simulink model "practical_class_2_2b_simulink"  (R2023b)
settings: Solver=VariableStepAuto  StartTime=0.0  StopTime=30  RelTol=1e-3
values from neighbouring files (symbols this model uses):
  b1 = 8    [practical_class_2_2b.m]
  b2 = 7    [practical_class_2_2b.m]
  k1 = 2    [practical_class_2_2b.m]
  k2 = 4    [practical_class_2_2b.m]
  m1 = 4    [practical_class_2_2b.m]
  m2 = 2    [practical_class_2_2b.m]
settings Model: Creator=klysm  LastModifiedBy=klysm

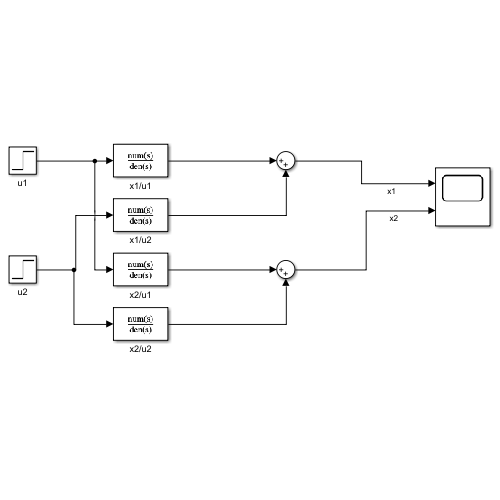
[thumbnail: Simulink's stored preview of the top-level diagram]
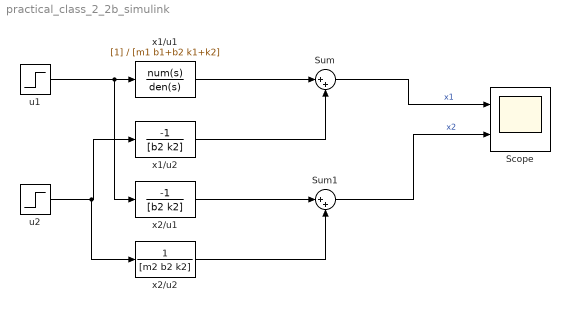
== system practical_class_2_2b_simulink ==
  Scope : Scope  NumInputPorts=2
  Sum : Sum  Inputs=|++
  Sum1 : Sum  Inputs=|++
  u1 : Step  Time=2  SampleTime=0
  u2 : Step  Time=10  After=0.7  SampleTime=0
  x1/u1 : TransferFcn  Denominator=[m1 b1+b2 k1+k2]
  x1/u2 : TransferFcn  Numerator=[-1]  Denominator=[b2 k2]
  x2/u1 : TransferFcn  Numerator=[-1]  Denominator=[b2 k2]
  x2/u2 : TransferFcn  Denominator=[m2 b2 k2]
  wires:
  Sum/1 -> Scope/1  "x1"
  Sum1/1 -> Scope/2  "x2"
  u1/1 -> x2/u1/1, x1/u1/1
  u2/1 -> x2/u2/1, x1/u2/1
  x1/u1/1 -> Sum/1
  x1/u2/1 -> Sum/2
  x2/u1/1 -> Sum1/1
  x2/u2/1 -> Sum1/2
